simulink model "lqg_demo"  (Simulink 6.0)
settings: Solver=ode45  SolverMode=SingleTasking  StartTime=0.0  StopTime=10  RelTol=1e-3  AbsTol=1e-6
PreLoadFcn:
  | load lqg_demo
values from neighbouring files (symbols this model uses):
  a = [-1.0285 -1.2903 0.1871 0.4069 0.9853 -1.0957 -3.8184 -4.1636 -0.9413 2.8689 -2.0788 2.5407 ... (16 elements, 4x4)]    [lqg_demo.mat]
  ae = [-0.450539168895 7.79314388558 -2.30165333018 -2.09634968553 0.61517890103 -6.91265861109 -2.22462397218 -2.56054063206 -0.9413 2.8689 -2.0788 2.5407 ... (16 elements, 4x4)]    [lqg_demo.mat]
  b = [0 6.6389 0 0]    [lqg_demo.mat]
  be = [0  0.324952676884; 6.6389  5.10707516338; 0  -1.39927658281; 0  -1.40742701312]    [lqg_demo.mat]
  c = [-1.7786 1.139 0 -1.0294]    [lqg_demo.mat]
  ce = [1 0 0 0 0 1 0 0 0 0 1 0 ... (16 elements, 4x4)]    [lqg_demo.mat]
  d = 0    [lqg_demo.mat]
  de = [0  0; 0  0; 0  0; 0  0]    [lqg_demo.mat]
  FF = 1    [lqg_demo.mat]
  K = [-1 1 0 -0.433 0.1]    [lqg_demo.mat]    (also in missile_demo.mat = [0.0258747790983 0.0212401146529 0.0177718187208 0.015129094)
libraries: srolib x1, simulink x1
settings Model: Creator=pascal  LastModifiedBy=pascal  ExtModeTrigMode=oneshot
settings DataIOCC: LimitDataPoints=off  SaveOutput=off  SaveTime=off  TimeSaveName=t  OutputSaveName=y  SignalLoggingName=logsOut
settings OptimizationCC: BooleanDataType=off
settings DebuggingCC: ConsistencyChecking=warning  CheckExecutionContextPreStartOutputMsg=on  CheckExecutionContextRuntimeOutputMsg=on  SolverPrmCheckMsg=none
settings HardwareCC: TargetUnknown=on
settings ModelReferenceCC: UpdateModelReferenceTargets=IfOutOfDate
settings GRTTargetCC: ModelReferenceCompliant=off
settings SFSimCC: SFSimApplyToAllLibs=on  SFSimBuildMode=Incremental

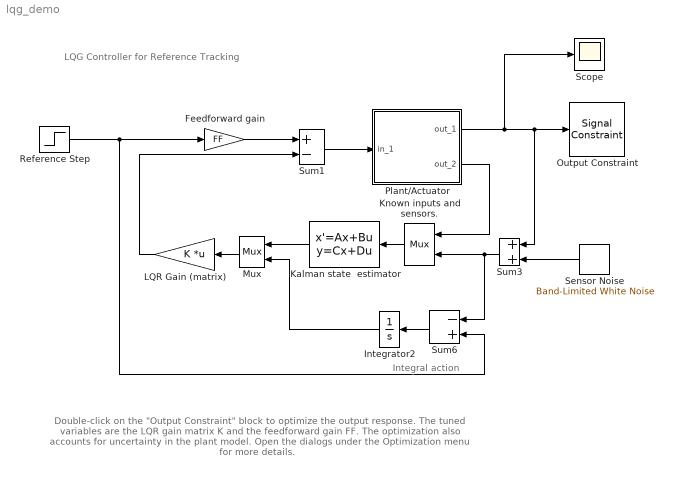
== system lqg_demo ==
  note: Double-click on the "Output Constraint" block to
      | optimize the output response.
      |
      | The tuned variables are the LQR gain matrix K and the feedforward gain FF.
      |  The optimization also accounts for uncertainty in the plant model.
      | Open the dialogs under the Optimization menu for more details.
  note: Integral action
  note: LQG Controller for Reference Tracking
  Feedforward gain : Gain  Gain=FF  SaturateOnIntegerOverflow=on
  Integrator2 : Integrator  Orientation=left
  Kalman state  estimator : StateSpace  Orientation=left  A=ae  B=be  C=ce  D=de
  Known inputs and sensors. : Mux  Orientation=left  Inputs=[1,1]
  LQR Gain (matrix) : Gain  Orientation=left  Gain=K  Multiplication=Matrix(K*u)
  Mux : Mux  Orientation=left  Inputs=[4,1]
  Output Constraint : srolib/Signal Constraint  DialogPosition=[0.063125 0.2675 0.36375 0.274166666666667]  SaveIn=workspace  SaveAs=lqg_optim  LogID=SRO_DataLog_1  Ylim=[-0.2 1.6]
  Plant/Actuator : Subsystem  PropExecContextAcrossSSBoundary=on
  Reference Step : Step  SampleTime=0
  Scope : Scope
  Sensor Noise : simulink/Sources/Band-Limited White Noise  Orientation=left  Cov=1e-5  Ts=0.1  seed=[23341]
  Sum1 : Sum  Inputs=+-  SaturateOnIntegerOverflow=on  InputSameDT=on
  Sum3 : Sum  Orientation=left  SaturateOnIntegerOverflow=on  InputSameDT=on
  Sum6 : Sum  Orientation=left  Inputs=-+  SaturateOnIntegerOverflow=on  InputSameDT=on
  wires:
  Reference Step/1 -> Sum6/2, Feedforward gain/1
  Feedforward gain/1 -> Sum1/1
  LQR Gain (matrix)/1 -> Sum1/2
  Sensor Noise/1 -> Sum3/2
  Sum3/1 -> Sum6/1, Known inputs and sensors./2
  Plant/Actuator/2(out_2) -> Known inputs and sensors./1
  Sum1/1 -> Plant/Actuator/1(in_1)
  Integrator2/1 -> Mux/2
  Sum6/1 -> Integrator2/1
  Known inputs and sensors./1 -> Kalman state  estimator/1
  Mux/1 -> LQR Gain (matrix)/1
  Kalman state  estimator/1 -> Mux/1
  Plant/Actuator/1(out_1) -> Output Constraint/1, Sum3/1, Scope/1

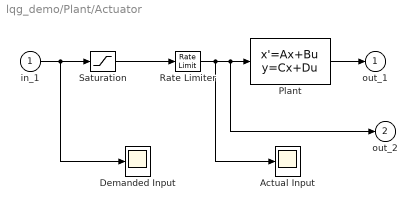
== system lqg_demo/Plant/Actuator ==
  in_1 : Inport  LatchInput=off
  "Actual Input " : Scope
      settings: TickLabels=on  TimeRange=10.100000  YMin=-3.000000  YMax=3.000000  DataFormat=Array
  "Demanded Input " : Scope
      settings: TickLabels=on  TimeRange=10.100000  YMin=-3.000000  YMax=3.000000  DataFormat=Array
  Plant : StateSpace  A=a  B=b  C=c  D=d
  Rate Limiter : RateLimiter  RisingSlewLimit=10  FallingSlewLimit=-10
  Saturation : Saturate  UpperLimit=5  LowerLimit=-5
  out_1 : Outport  InitialOutput=0
  out_2 : Outport  Port=2  InitialOutput=0
  wires:
  Rate Limiter/1 -> "Actual Input "/1, out_2/1, Plant/1
  in_1/1 -> "Demanded Input "/1, Saturation/1
  Plant/1 -> out_1/1
  Saturation/1 -> Rate Limiter/1
